simulink model "DemonstratorSimscape"  (R2020b)
settings: Solver=ode113  StartTime=0.0  StopTime=t_stop*0+20  FixedStep=1e-4
values from neighbouring files (symbols this model uses):
  brkD = 0    [main.m]
  brkI = 1e4    (= 10000)    [main.m]
  brkP = 1e5    (= 100000)    [main.m]
  d_drm = 0.5*d_drum    [main.m]
  d_shm = 0.4*d_sheave    [main.m]
  DeltaCable0 = 0    [main.m]
  Droop_scaling = 0    [main.m]
  eta_sh = 0.015    [main.m]
  filt_NUM = ones(1,200)*0.005    [main.m]
  g = 9.80665    [main.m]
  Iw = 0.5*(W.i + M.in*GB.r^2)    [main.m]
  Kp_mul = 0.3    [main.m]
  Lc0 = abs((T.ph-L.height-P.d-L.z0)*0.001)    [main.m]
  Ls1 = ((T.ph-0.5*W.pd)/1000)    [main.m]
  Ls2 = ((0.5*(T.s2+P.d)-2*P.d)/1000)    [main.m]
  M = 50e3    (= 50000)    [calcGrav.m]
  phi0_drm = -90    [main.m]
  phi0_shm = -90    [main.m]
  r_sheave = P.d*0.5    [main.m]
  s = tf('s')    [calcGrav.m]
  tau_brk = 0.001    [main.m]
  tau_em = 60e-3    (= 0.06)    [calcGrav.m]    (also in main.m)
  tau_m = tau_w/GB.r    [main.m]
  Tmax = 400e3    (= 400000)    [main.m]
  Tn_mul = 10    [main.m]
  x_drm = 0.7*r_drum    [main.m]
  x_shm = 0.7*r_sheave    [main.m]
  z0 = 0    [calcGrav.m]    (also in main.m = L.z0-P.d*0.5-P.d-P.d-L.height-T.h1-T.h2-32)
undefined symbols (not defined in the file or in its folder): C, CA, Controller_sampleTime, DiscIntNeverNeededParam, GB, L, P, Part, T, VFD_acceleration_model_factor, VFD_Adapt_factor_lower_p1458, VFD_Adapt_factor_upper_p1459, VFD_Curr_limit_var_p0641, VFD_Current_limit_p0640, VFD_Id_setp_total_r1624, VFD_Iq, VFD_Kp_n_basic_p1460, VFD_M, VFD_M_accel_T_smooth_p1517, VFD_M_lim_var_fixS_src_p1551, VFD_M_max_lower_p1521, VFD_M_max_lower_scal_p1525, VFD_M_max_up_mot_scal_p1524, VFD_M_max_upper_p1520, VFD_n_act_T_smooth_p1442, VFD_n_ctr_Kp_n_up_scal_p1461, VFD_n_ctr_Tn_n_up_sca_p1463, VFD_n_ctrl_adapt_Kp_lower_p1456, VFD_n_ctrl_adapt_Kp_upper_p1457, VFD_n_ctrl_Adpt_sig_Kp_p1455, VFD_n_ctrl_Kp_scal_p1466, VFD_n_ctrl_n_lower_p1464, VFD_n_ctrl_n_upper_p1465, VFD_n_ctrl_Tn_n_lower_p1462, VFD_n_limit_neg_p1086, VFD_n_limit_pos_p1083, VFD_n_limit_setp_p1063, VFD_n_max_p1082, VFD_n_set_filt_1_T_p1416, VFD_P_max_gen_p1531, VFD_P_max_mot_p1530, VFD_PU_I_outp_max_r0289, VFD_RFG_ramp_down_time_p1121, VFD_RFG_ramp_up_time_p1120, VFD_RFG_t_RD_scal_p1139, VFD_RFG_t_RU_scal_p1138, VSD, W, X, Y, Z
libraries: sm_lib x248, nesl_utility x128, simulink x49, pid_lib x4, cstblocks x2, simulink_extras x2
(part 7 of 10)

== system DemonstratorSimscape/Transmission System/Anchor and Load/Sheave_03/Sheave3 ==
  Rigid Transform : sm_lib/Frames and Transforms/Rigid Transform  TranslationMethod=None  TranslationStandardOffset=0  TranslationLengthUnit=m  TranslationStandardAxis=+Z  TranslationCartesianOffset=[0 0 0]  TranslationROffset=0  TranslationROffsetUnits=m  TranslationZOffset=0  TranslationZOffsetUnits=m  TranslationThetaOffset=0  TranslationThetaOffsetUnits=deg  RotationMethod=StandardAxis  RotationAngleUnits=deg  RotationStandardAxis=+X  RotationAngle=90  RotationArbitraryAxis=[0 0 1]  FollAlignAxisA=+X  BaseAlignAxisA=+Y  FollAlignAxisB=+Y  BaseAlignAxisB=+Z  RotationSequenceAxes=FollowerAxes  RotationSequence=XYX  RotationSequenceAngles=[0 0 0]  RotationSequenceAnglesUnits=deg  RotationMatrix=[1 0 0; 0 1 0; 0 0 1]
  pulley1 : sm_lib/Body Elements/Cylindrical Solid  GraphicAmbientColor=[0.15 0.15 0.15 1.0]  BasedOnType=Mass  CenterOfMass=[0 0 0]  CenterOfMassUnits=m  GraphicDiffuseColor=c.sheave  CylinderLength=P.h  CylinderLengthUnits=mm  CylinderRadius=P.d*0.5  CylinderRadiusUnits=mm  Density=0  DensityUnits=kg/m^3  DoExposeReferenceFrame=off  GraphicEmissiveColor=[0.0 0.0 0.0 1.0]  ExportEntireGeometry=off  SerializedFrames=<Frames><Frame><Id>Frame1</Id><Value><Name>F1</Name><Origin><Source>ReferenceFrame</Source><FeatureName></FeatureName></Origin><PrimaryAxis><DefinedDirection>+Z</DefinedDirection><Source>ReferenceFrame</Source><SourceDirection>-Y</SourceDirection><FeatureName></FeatureName></PrimaryAxis><SecondaryAxis><DefinedDirection>+X</DefinedDirection><Source>ReferenceFrame</Source><SourceDirection>+X</SourceDirection><FeatureName></FeatureName></SecondaryAxis></Value></Frame></Frames>  MarkerShape=Frame  MarkerSize=10  GraphicType=FromGeometry  InertiaType=CalculateFromGeometry  Mass=P.m  MassUnits=kg  MomentsOfInertia=[1 1 1]  MomentsOfInertiaUnits=kg*m^2  GraphicOpacity=1.0  ProductsOfInertia=[0 0 0]  ProductsOfInertiaUnits=kg*m^2  GraphicShininess=10  GraphicSpecularColor=[0.8 0.8 0.8]  GraphicVisPropType=SimpleVisualProperties
  tags : Subsystem  mask{phi0=phi0_shm, s=-1}
      mask prompts: phi0 "angle (deg)"; s "direction (1 | -1)"
  F : PMIOPort  Side=Left
  R : PMIOPort  Port=2  Side=Right
  connections:
  R/RConn1 -- tags/LConn1 -- Rigid Transform/RConn1 -- F/RConn1
  pulley1/LConn1 -- Rigid Transform/LConn1

== system DemonstratorSimscape/Transmission System/Anchor and Load/Sheave_05/Bending loss ==
  Sin (kN) : Inport
  w (deg/s) : Inport  Port=2
  Add : Sum
  Add1 : Sum  Inputs=+-
  Constant : Constant
  Constant2 : Constant
  Math Function : Math  Operator=pow  SignedPower=on  SaturateOnIntegerOverflow=on
  Product : Product
  Product1 : Product
  Scope : Scope
  dT_Gain : Gain  Gain=0
  dr for positive omega : Constant  Value=-1
  dr switch : MATLAB Function  TreatAsAtomicUnit=on
  eta_sh : Constant  Value=eta_sh
  torque (Nm) : Gain  Gain=r_sheave
  dT (Nm) : Outport  VectorParamsAs1DForOutWhenUnconnected=off
  Sout (kN) : Outport  Port=2  VectorParamsAs1DForOutWhenUnconnected=off
  wires:
  Add/1 -> Math Function/1
  Sin (kN)/1 -> Product1/2, Product/2
  torque (Nm)/1 -> Scope/1, dT_Gain/1
  Math Function/1 -> Add1/1, Product1/1
  Add1/1 -> Product/1
  Product/1 -> torque (Nm)/1
  eta_sh/1 -> Add/2
  Constant/1 -> Add/1
  Constant2/1 -> Add1/2
  Product1/1 -> Sout (kN)/1
  dT_Gain/1 -> dT (Nm)/1
  dr for positive omega/1 -> dr switch/2(dr_wpos)
  dr switch/1(dr) -> Math Function/2
  w (deg/s)/1 -> dr switch/1(w)

== system DemonstratorSimscape/Transmission System/Anchor and Load/Sheave_05/PS>Sim2 ==
  b (deg/s^2) : nesl_utility/PS-Simulink Converter  PhysicalDomain=network_engine_domain  SubClassName=ps_output  LeftPortType=input  RightPortType=output  PseudoPeriodic=off  Frequencies=[]  Unit=deg/s^2  AffineConversion=off
  fc (N) : nesl_utility/PS-Simulink Converter  PhysicalDomain=network_engine_domain  SubClassName=ps_output  LeftPortType=input  RightPortType=output  PseudoPeriodic=off  Frequencies=[]  Unit=N  AffineConversion=off
  ft (N) : nesl_utility/PS-Simulink Converter  PhysicalDomain=network_engine_domain  SubClassName=ps_output  LeftPortType=input  RightPortType=output  PseudoPeriodic=off  Frequencies=[]  Unit=N  AffineConversion=off
  q (deg) : nesl_utility/PS-Simulink Converter  PhysicalDomain=network_engine_domain  SubClassName=ps_output  LeftPortType=input  RightPortType=output  PseudoPeriodic=off  Frequencies=[]  Unit=deg  AffineConversion=off
  t (Nm) : nesl_utility/PS-Simulink Converter  PhysicalDomain=network_engine_domain  SubClassName=ps_output  LeftPortType=input  RightPortType=output  PseudoPeriodic=off  Frequencies=[]  Unit=N*m  AffineConversion=off
  tc (Nm) : nesl_utility/PS-Simulink Converter  PhysicalDomain=network_engine_domain  SubClassName=ps_output  LeftPortType=input  RightPortType=output  PseudoPeriodic=off  Frequencies=[]  Unit=N*m  AffineConversion=off
  tt (Nm) : nesl_utility/PS-Simulink Converter  PhysicalDomain=network_engine_domain  SubClassName=ps_output  LeftPortType=input  RightPortType=output  PseudoPeriodic=off  Frequencies=[]  Unit=N*m  AffineConversion=off
  w (deg/s) : nesl_utility/PS-Simulink Converter  PhysicalDomain=network_engine_domain  SubClassName=ps_output  LeftPortType=input  RightPortType=output  PseudoPeriodic=off  Frequencies=[]  Unit=deg/s  AffineConversion=off
  q : PMIOPort  Side=Left
  Conn2 : PMIOPort  Port=2  Side=Left
  Conn3 : PMIOPort  Port=3  Side=Left
  Conn4 : PMIOPort  Port=4  Side=Left
  Conn5 : PMIOPort  Port=5  Side=Left
  Conn6 : PMIOPort  Port=6  Side=Left
  Conn7 : PMIOPort  Port=7  Side=Left
  Conn8 : PMIOPort  Port=8  Side=Left
  Out1 : Outport  VectorParamsAs1DForOutWhenUnconnected=off
  Out2 : Outport  Port=2  VectorParamsAs1DForOutWhenUnconnected=off
  Out3 : Outport  Port=3  VectorParamsAs1DForOutWhenUnconnected=off
  Out4 : Outport  Port=4  VectorParamsAs1DForOutWhenUnconnected=off
  Out5 : Outport  Port=5  VectorParamsAs1DForOutWhenUnconnected=off
  Out6 : Outport  Port=6  VectorParamsAs1DForOutWhenUnconnected=off
  Out7 : Outport  Port=7  VectorParamsAs1DForOutWhenUnconnected=off
  Out8 : Outport  Port=8  VectorParamsAs1DForOutWhenUnconnected=off
  wires:
  tt (Nm)/1 -> Out8/1
  ft (N)/1 -> Out7/1
  tc (Nm)/1 -> Out6/1
  fc (N)/1 -> Out5/1
  t (Nm)/1 -> Out4/1
  b (deg/s^2)/1 -> Out3/1
  w (deg/s)/1 -> Out2/1
  q (deg)/1 -> Out1/1
  connections:
  Conn8/RConn1 -- tt (Nm)/LConn1
  ft (N)/LConn1 -- Conn7/RConn1
  Conn6/RConn1 -- tc (Nm)/LConn1
  fc (N)/LConn1 -- Conn5/RConn1
  Conn4/RConn1 -- t (Nm)/LConn1
  Conn3/RConn1 -- b (deg/s^2)/LConn1
  Conn2/RConn1 -- w (deg/s)/LConn1
  q/RConn1 -- q (deg)/LConn1

== system DemonstratorSimscape/Transmission System/Anchor and Load/Sheave_05/Sheave5 ==
  Rigid Transform : sm_lib/Frames and Transforms/Rigid Transform  TranslationMethod=None  TranslationStandardOffset=0  TranslationLengthUnit=m  TranslationStandardAxis=+Z  TranslationCartesianOffset=[0 0 0]  TranslationROffset=0  TranslationROffsetUnits=m  TranslationZOffset=0  TranslationZOffsetUnits=m  TranslationThetaOffset=0  TranslationThetaOffsetUnits=deg  RotationMethod=StandardAxis  RotationAngleUnits=deg  RotationStandardAxis=+X  RotationAngle=90  RotationArbitraryAxis=[0 0 1]  FollAlignAxisA=+X  BaseAlignAxisA=+Y  FollAlignAxisB=+Y  BaseAlignAxisB=+Z  RotationSequenceAxes=FollowerAxes  RotationSequence=XYX  RotationSequenceAngles=[0 0 0]  RotationSequenceAnglesUnits=deg  RotationMatrix=[1 0 0; 0 1 0; 0 0 1]
  pulley2 : sm_lib/Body Elements/Cylindrical Solid  GraphicAmbientColor=[0.15 0.15 0.15 1.0]  BasedOnType=Mass  CenterOfMass=[0 0 0]  CenterOfMassUnits=m  GraphicDiffuseColor=c.sheave  CylinderLength=P.h  CylinderLengthUnits=mm  CylinderRadius=P.d*0.5  CylinderRadiusUnits=mm  Density=0  DensityUnits=kg/m^3  DoExposeReferenceFrame=off  GraphicEmissiveColor=[0.0 0.0 0.0 1.0]  ExportEntireGeometry=off  SerializedFrames=<Frames><Frame><Id>Frame1</Id><Value><Name>F1</Name><Origin><Source>ReferenceFrame</Source><FeatureName></FeatureName></Origin><PrimaryAxis><DefinedDirection>+Z</DefinedDirection><Source>ReferenceFrame</Source><SourceDirection>-Y</SourceDirection><FeatureName></FeatureName></PrimaryAxis><SecondaryAxis><DefinedDirection>+X</DefinedDirection><Source>ReferenceFrame</Source><SourceDirection>+X</SourceDirection><FeatureName></FeatureName></SecondaryAxis></Value></Frame></Frames>  MarkerShape=Frame  MarkerSize=10  GraphicType=FromGeometry  InertiaType=CalculateFromGeometry  Mass=P.m  MassUnits=kg  MomentsOfInertia=[1 1 1]  MomentsOfInertiaUnits=kg*m^2  GraphicOpacity=1.0  ProductsOfInertia=[0 0 0]  ProductsOfInertiaUnits=kg*m^2  GraphicShininess=10  GraphicSpecularColor=[0.8 0.8 0.8]  GraphicVisPropType=SimpleVisualProperties
  tags : Subsystem  mask{phi0=phi0_shm, s=-1}
      mask prompts: phi0 "angle (deg)"; s "direction (1 | -1)"
  F : PMIOPort  Side=Left
  R : PMIOPort  Port=2  Side=Right
  connections:
  R/RConn1 -- tags/LConn1 -- Rigid Transform/RConn1 -- F/RConn1
  pulley2/LConn1 -- Rigid Transform/LConn1

== system DemonstratorSimscape/Transmission System/Roof Pulley Set/Sheave_01/Bending loss ==
  Sin (kN) : Inport
  w (deg/s) : Inport  Port=2
  Add : Sum
  Add1 : Sum  Inputs=+-
  Constant : Constant
  Constant2 : Constant
  Math Function : Math  Operator=pow  SignedPower=on  SaturateOnIntegerOverflow=on
  Product : Product
  Product1 : Product
  Scope : Scope
  dT_Gain : Gain
  dr for positive omega : Constant  Value=-1
  dr switch : MATLAB Function  TreatAsAtomicUnit=on
  eta_sh : Constant  Value=eta_sh/2
  torque (Nm) : Gain  Gain=r_sheave
  dT (Nm) : Outport  VectorParamsAs1DForOutWhenUnconnected=off
  Sout (kN) : Outport  Port=2  VectorParamsAs1DForOutWhenUnconnected=off
  wires:
  Add/1 -> Math Function/1
  Sin (kN)/1 -> Product1/2, Product/2
  torque (Nm)/1 -> Scope/1, dT_Gain/1
  Math Function/1 -> Add1/1, Product1/1
  Add1/1 -> Product/1
  Product/1 -> torque (Nm)/1
  eta_sh/1 -> Add/2
  Constant/1 -> Add/1
  Constant2/1 -> Add1/2
  Product1/1 -> Sout (kN)/1
  dT_Gain/1 -> dT (Nm)/1
  dr for positive omega/1 -> dr switch/2(dr_wpos)
  dr switch/1(dr) -> Math Function/2
  w (deg/s)/1 -> dr switch/1(w)

== system DemonstratorSimscape/Transmission System/Roof Pulley Set/Sheave_01/PS>Sim1 ==
  b (deg/s^2) : nesl_utility/PS-Simulink Converter  PhysicalDomain=network_engine_domain  SubClassName=ps_output  LeftPortType=input  RightPortType=output  PseudoPeriodic=off  Frequencies=[]  Unit=deg/s^2  AffineConversion=off
  fc (N) : nesl_utility/PS-Simulink Converter  PhysicalDomain=network_engine_domain  SubClassName=ps_output  LeftPortType=input  RightPortType=output  PseudoPeriodic=off  Frequencies=[]  Unit=N  AffineConversion=off
  ft (N) : nesl_utility/PS-Simulink Converter  PhysicalDomain=network_engine_domain  SubClassName=ps_output  LeftPortType=input  RightPortType=output  PseudoPeriodic=off  Frequencies=[]  Unit=N  AffineConversion=off
  q (deg) : nesl_utility/PS-Simulink Converter  PhysicalDomain=network_engine_domain  SubClassName=ps_output  LeftPortType=input  RightPortType=output  PseudoPeriodic=off  Frequencies=[]  Unit=deg  AffineConversion=off
  t (Nm) : nesl_utility/PS-Simulink Converter  PhysicalDomain=network_engine_domain  SubClassName=ps_output  LeftPortType=input  RightPortType=output  PseudoPeriodic=off  Frequencies=[]  Unit=N*m  AffineConversion=off
  tc (Nm) : nesl_utility/PS-Simulink Converter  PhysicalDomain=network_engine_domain  SubClassName=ps_output  LeftPortType=input  RightPortType=output  PseudoPeriodic=off  Frequencies=[]  Unit=N*m  AffineConversion=off
  tt (Nm) : nesl_utility/PS-Simulink Converter  PhysicalDomain=network_engine_domain  SubClassName=ps_output  LeftPortType=input  RightPortType=output  PseudoPeriodic=off  Frequencies=[]  Unit=N*m  AffineConversion=off
  w (deg/s) : nesl_utility/PS-Simulink Converter  PhysicalDomain=network_engine_domain  SubClassName=ps_output  LeftPortType=input  RightPortType=output  PseudoPeriodic=off  Frequencies=[]  Unit=deg/s  AffineConversion=off
  q : PMIOPort  Side=Left
  Conn2 : PMIOPort  Port=2  Side=Left
  Conn3 : PMIOPort  Port=3  Side=Left
  Conn4 : PMIOPort  Port=4  Side=Left
  Conn5 : PMIOPort  Port=5  Side=Left
  Conn6 : PMIOPort  Port=6  Side=Left
  Conn7 : PMIOPort  Port=7  Side=Left
  Conn8 : PMIOPort  Port=8  Side=Left
  Out1 : Outport  VectorParamsAs1DForOutWhenUnconnected=off
  Out2 : Outport  Port=2  VectorParamsAs1DForOutWhenUnconnected=off
  Out3 : Outport  Port=3  VectorParamsAs1DForOutWhenUnconnected=off
  Out4 : Outport  Port=4  VectorParamsAs1DForOutWhenUnconnected=off
  Out5 : Outport  Port=5  VectorParamsAs1DForOutWhenUnconnected=off
  Out6 : Outport  Port=6  VectorParamsAs1DForOutWhenUnconnected=off
  Out7 : Outport  Port=7  VectorParamsAs1DForOutWhenUnconnected=off
  Out8 : Outport  Port=8  VectorParamsAs1DForOutWhenUnconnected=off
  wires:
  q (deg)/1 -> Out1/1
  w (deg/s)/1 -> Out2/1
  b (deg/s^2)/1 -> Out3/1
  t (Nm)/1 -> Out4/1
  fc (N)/1 -> Out5/1
  tc (Nm)/1 -> Out6/1
  ft (N)/1 -> Out7/1
  tt (Nm)/1 -> Out8/1
  connections:
  q/RConn1 -- q (deg)/LConn1
  Conn2/RConn1 -- w (deg/s)/LConn1
  Conn3/RConn1 -- b (deg/s^2)/LConn1
  Conn4/RConn1 -- t (Nm)/LConn1
  fc (N)/LConn1 -- Conn5/RConn1
  Conn6/RConn1 -- tc (Nm)/LConn1
  ft (N)/LConn1 -- Conn7/RConn1
  Conn8/RConn1 -- tt (Nm)/LConn1

== system DemonstratorSimscape/Transmission System/Roof Pulley Set/Sheave_01/Sheave1 ==
  Rigid Transform : sm_lib/Frames and Transforms/Rigid Transform  TranslationMethod=None  TranslationStandardOffset=0  TranslationLengthUnit=m  TranslationStandardAxis=+Z  TranslationCartesianOffset=[0 0 0]  TranslationROffset=0  TranslationROffsetUnits=m  TranslationZOffset=0  TranslationZOffsetUnits=m  TranslationThetaOffset=0  TranslationThetaOffsetUnits=deg  RotationMethod=StandardAxis  RotationAngleUnits=deg  RotationStandardAxis=+X  RotationAngle=90  RotationArbitraryAxis=[0 0 1]  FollAlignAxisA=+X  BaseAlignAxisA=+Y  FollAlignAxisB=+Y  BaseAlignAxisB=+Z  RotationSequenceAxes=FollowerAxes  RotationSequence=XYX  RotationSequenceAngles=[0 0 0]  RotationSequenceAnglesUnits=deg  RotationMatrix=[1 0 0; 0 1 0; 0 0 1]
  pulley2 : sm_lib/Body Elements/Cylindrical Solid  GraphicAmbientColor=[0.15 0.15 0.15 1.0]  BasedOnType=Mass  CenterOfMass=[0 0 0]  CenterOfMassUnits=m  GraphicDiffuseColor=c.sheave  CylinderLength=P.h  CylinderLengthUnits=mm  CylinderRadius=P.d*0.5  CylinderRadiusUnits=mm  Density=L.den  DensityUnits=g/cm^3  DoExposeReferenceFrame=off  GraphicEmissiveColor=[0.0 0.0 0.0 1.0]  ExportEntireGeometry=off  SerializedFrames=<Frames><Frame><Id>Frame1</Id><Value><Name>F1</Name><Origin><Source>ReferenceFrame</Source><FeatureName></FeatureName></Origin><PrimaryAxis><DefinedDirection>+Z</DefinedDirection><Source>ReferenceFrame</Source><SourceDirection>-Y</SourceDirection><FeatureName></FeatureName></PrimaryAxis><SecondaryAxis><DefinedDirection>+X</DefinedDirection><Source>ReferenceFrame</Source><SourceDirection>+X</SourceDirection><FeatureName></FeatureName></SecondaryAxis></Value></Frame></Frames>  MarkerShape=Frame  MarkerSize=10  GraphicType=FromGeometry  InertiaType=CalculateFromGeometry  Mass=P.m  MassUnits=kg  MomentsOfInertia=[1 1 1]  MomentsOfInertiaUnits=kg*m^2  GraphicOpacity=1.0  ProductsOfInertia=[0 0 0]  ProductsOfInertiaUnits=kg*m^2  GraphicShininess=10  GraphicSpecularColor=[0.8 0.8 0.8]  GraphicVisPropType=SimpleVisualProperties
  tags : Subsystem  mask{phi0=phi0_shm, s=1}
      mask prompts: phi0 "angle (deg)"; s "direction (1 | -1)"
  F : PMIOPort  Side=Left
  R : PMIOPort  Port=2  Side=Right
  connections:
  R/RConn1 -- tags/LConn1 -- Rigid Transform/RConn1 -- F/RConn1
  pulley2/LConn1 -- Rigid Transform/LConn1

== system DemonstratorSimscape/Transmission System/Roof Pulley Set/Sheave_02/Bending loss ==
  Sin (kN) : Inport
  w (deg/s) : Inport  Port=2
  Add : Sum
  Add1 : Sum  Inputs=+-
  Constant : Constant
  Constant2 : Constant
  Math Function : Math  Operator=pow  SignedPower=on  SaturateOnIntegerOverflow=on
  Product : Product
  Product1 : Product
  Scope : Scope
  dT_Gain : Gain
  dr for positive omega : Constant  Value=-1
  dr switch : MATLAB Function  TreatAsAtomicUnit=on
  eta_sh : Constant  Value=eta_sh/2
  torque (Nm) : Gain  Gain=r_sheave
  dT (Nm) : Outport  VectorParamsAs1DForOutWhenUnconnected=off
  Sout (kN) : Outport  Port=2  VectorParamsAs1DForOutWhenUnconnected=off
  wires:
  Add/1 -> Math Function/1
  Sin (kN)/1 -> Product1/2, Product/2
  torque (Nm)/1 -> Scope/1, dT_Gain/1
  Math Function/1 -> Add1/1, Product1/1
  Add1/1 -> Product/1
  Product/1 -> torque (Nm)/1
  eta_sh/1 -> Add/2
  Constant/1 -> Add/1
  Constant2/1 -> Add1/2
  Product1/1 -> Sout (kN)/1
  dT_Gain/1 -> dT (Nm)/1
  dr for positive omega/1 -> dr switch/2(dr_wpos)
  dr switch/1(dr) -> Math Function/2
  w (deg/s)/1 -> dr switch/1(w)

== system DemonstratorSimscape/Transmission System/Roof Pulley Set/Sheave_02/PS>Sim1 ==
  b (deg/s^2) : nesl_utility/PS-Simulink Converter  PhysicalDomain=network_engine_domain  SubClassName=ps_output  LeftPortType=input  RightPortType=output  PseudoPeriodic=off  Frequencies=[]  Unit=deg/s^2  AffineConversion=off
  fc (N) : nesl_utility/PS-Simulink Converter  PhysicalDomain=network_engine_domain  SubClassName=ps_output  LeftPortType=input  RightPortType=output  PseudoPeriodic=off  Frequencies=[]  Unit=N  AffineConversion=off
  ft (N) : nesl_utility/PS-Simulink Converter  PhysicalDomain=network_engine_domain  SubClassName=ps_output  LeftPortType=input  RightPortType=output  PseudoPeriodic=off  Frequencies=[]  Unit=N  AffineConversion=off
  q (deg) : nesl_utility/PS-Simulink Converter  PhysicalDomain=network_engine_domain  SubClassName=ps_output  LeftPortType=input  RightPortType=output  PseudoPeriodic=off  Frequencies=[]  Unit=deg  AffineConversion=off
  t (Nm) : nesl_utility/PS-Simulink Converter  PhysicalDomain=network_engine_domain  SubClassName=ps_output  LeftPortType=input  RightPortType=output  PseudoPeriodic=off  Frequencies=[]  Unit=N*m  AffineConversion=off
  tc (Nm) : nesl_utility/PS-Simulink Converter  PhysicalDomain=network_engine_domain  SubClassName=ps_output  LeftPortType=input  RightPortType=output  PseudoPeriodic=off  Frequencies=[]  Unit=N*m  AffineConversion=off
  tt (Nm) : nesl_utility/PS-Simulink Converter  PhysicalDomain=network_engine_domain  SubClassName=ps_output  LeftPortType=input  RightPortType=output  PseudoPeriodic=off  Frequencies=[]  Unit=N*m  AffineConversion=off
  w (deg/s) : nesl_utility/PS-Simulink Converter  PhysicalDomain=network_engine_domain  SubClassName=ps_output  LeftPortType=input  RightPortType=output  PseudoPeriodic=off  Frequencies=[]  Unit=deg/s  AffineConversion=off
  q : PMIOPort  Side=Left
  Conn2 : PMIOPort  Port=2  Side=Left
  Conn3 : PMIOPort  Port=3  Side=Left
  Conn4 : PMIOPort  Port=4  Side=Left
  Conn5 : PMIOPort  Port=5  Side=Left
  Conn6 : PMIOPort  Port=6  Side=Left
  Conn7 : PMIOPort  Port=7  Side=Left
  Conn8 : PMIOPort  Port=8  Side=Left
  Out1 : Outport  VectorParamsAs1DForOutWhenUnconnected=off
  Out2 : Outport  Port=2  VectorParamsAs1DForOutWhenUnconnected=off
  Out3 : Outport  Port=3  VectorParamsAs1DForOutWhenUnconnected=off
  Out4 : Outport  Port=4  VectorParamsAs1DForOutWhenUnconnected=off
  Out5 : Outport  Port=5  VectorParamsAs1DForOutWhenUnconnected=off
  Out6 : Outport  Port=6  VectorParamsAs1DForOutWhenUnconnected=off
  Out7 : Outport  Port=7  VectorParamsAs1DForOutWhenUnconnected=off
  Out8 : Outport  Port=8  VectorParamsAs1DForOutWhenUnconnected=off
  wires:
  tt (Nm)/1 -> Out8/1
  ft (N)/1 -> Out7/1
  tc (Nm)/1 -> Out6/1
  fc (N)/1 -> Out5/1
  t (Nm)/1 -> Out4/1
  b (deg/s^2)/1 -> Out3/1
  w (deg/s)/1 -> Out2/1
  q (deg)/1 -> Out1/1
  connections:
  Conn8/RConn1 -- tt (Nm)/LConn1
  ft (N)/LConn1 -- Conn7/RConn1
  Conn6/RConn1 -- tc (Nm)/LConn1
  fc (N)/LConn1 -- Conn5/RConn1
  Conn4/RConn1 -- t (Nm)/LConn1
  Conn3/RConn1 -- b (deg/s^2)/LConn1
  Conn2/RConn1 -- w (deg/s)/LConn1
  q/RConn1 -- q (deg)/LConn1

== system DemonstratorSimscape/Transmission System/Roof Pulley Set/Sheave_02/Sheave2 ==
  Rigid Transform : sm_lib/Frames and Transforms/Rigid Transform  TranslationMethod=None  TranslationStandardOffset=0  TranslationLengthUnit=m  TranslationStandardAxis=+Z  TranslationCartesianOffset=[0 0 0]  TranslationROffset=0  TranslationROffsetUnits=m  TranslationZOffset=0  TranslationZOffsetUnits=m  TranslationThetaOffset=0  TranslationThetaOffsetUnits=deg  RotationMethod=StandardAxis  RotationAngleUnits=deg  RotationStandardAxis=+X  RotationAngle=90  RotationArbitraryAxis=[0 0 1]  FollAlignAxisA=+X  BaseAlignAxisA=+Y  FollAlignAxisB=+Y  BaseAlignAxisB=+Z  RotationSequenceAxes=FollowerAxes  RotationSequence=XYX  RotationSequenceAngles=[0 0 0]  RotationSequenceAnglesUnits=deg  RotationMatrix=[1 0 0; 0 1 0; 0 0 1]
  pulley2 : sm_lib/Body Elements/Cylindrical Solid  GraphicAmbientColor=[0.15 0.15 0.15 1.0]  BasedOnType=Mass  CenterOfMass=[0 0 0]  CenterOfMassUnits=m  GraphicDiffuseColor=c.sheave  CylinderLength=P.h  CylinderLengthUnits=mm  CylinderRadius=P.d*0.5  CylinderRadiusUnits=mm  Density=0  DensityUnits=kg/m^3  DoExposeReferenceFrame=off  GraphicEmissiveColor=[0.0 0.0 0.0 1.0]  ExportEntireGeometry=off  SerializedFrames=<Frames><Frame><Id>Frame1</Id><Value><Name>F1</Name><Origin><Source>ReferenceFrame</Source><FeatureName></FeatureName></Origin><PrimaryAxis><DefinedDirection>+Z</DefinedDirection><Source>ReferenceFrame</Source><SourceDirection>-Y</SourceDirection><FeatureName></FeatureName></PrimaryAxis><SecondaryAxis><DefinedDirection>+X</DefinedDirection><Source>ReferenceFrame</Source><SourceDirection>+X</SourceDirection><FeatureName></FeatureName></SecondaryAxis></Value></Frame></Frames>  MarkerShape=Frame  MarkerSize=10  GraphicType=FromGeometry  InertiaType=CalculateFromGeometry  Mass=P.m  MassUnits=kg  MomentsOfInertia=[1 1 1]  MomentsOfInertiaUnits=kg*m^2  GraphicOpacity=1.0  ProductsOfInertia=[0 0 0]  ProductsOfInertiaUnits=kg*m^2  GraphicShininess=10  GraphicSpecularColor=[0.8 0.8 0.8]  GraphicVisPropType=SimpleVisualProperties
  tags : Subsystem  mask{phi0=phi0_shm, s=1}
      mask prompts: phi0 "angle (deg)"; s "direction (1 | -1)"
  F : PMIOPort  Side=Left
  R : PMIOPort  Port=2  Side=Right
  connections:
  R/RConn1 -- Rigid Transform/RConn1 -- tags/LConn1 -- F/RConn1
  pulley2/LConn1 -- Rigid Transform/LConn1

== system DemonstratorSimscape/Transmission System/Roof Pulley Set/Sheave_04/PS>Sim1 ==
  b (deg/s^2) : nesl_utility/PS-Simulink Converter  PhysicalDomain=network_engine_domain  SubClassName=ps_output  LeftPortType=input  RightPortType=output  PseudoPeriodic=off  Frequencies=[]  Unit=deg/s^2  AffineConversion=off
  fc (N) : nesl_utility/PS-Simulink Converter  PhysicalDomain=network_engine_domain  SubClassName=ps_output  LeftPortType=input  RightPortType=output  PseudoPeriodic=off  Frequencies=[]  Unit=N  AffineConversion=off
  ft (N) : nesl_utility/PS-Simulink Converter  PhysicalDomain=network_engine_domain  SubClassName=ps_output  LeftPortType=input  RightPortType=output  PseudoPeriodic=off  Frequencies=[]  Unit=N  AffineConversion=off
  q (deg) : nesl_utility/PS-Simulink Converter  PhysicalDomain=network_engine_domain  SubClassName=ps_output  LeftPortType=input  RightPortType=output  PseudoPeriodic=off  Frequencies=[]  Unit=deg  AffineConversion=off
  t (Nm) : nesl_utility/PS-Simulink Converter  PhysicalDomain=network_engine_domain  SubClassName=ps_output  LeftPortType=input  RightPortType=output  PseudoPeriodic=off  Frequencies=[]  Unit=N*m  AffineConversion=off
  tc (Nm) : nesl_utility/PS-Simulink Converter  PhysicalDomain=network_engine_domain  SubClassName=ps_output  LeftPortType=input  RightPortType=output  PseudoPeriodic=off  Frequencies=[]  Unit=N*m  AffineConversion=off
  tt (Nm) : nesl_utility/PS-Simulink Converter  PhysicalDomain=network_engine_domain  SubClassName=ps_output  LeftPortType=input  RightPortType=output  PseudoPeriodic=off  Frequencies=[]  Unit=N*m  AffineConversion=off
  w (deg/s) : nesl_utility/PS-Simulink Converter  PhysicalDomain=network_engine_domain  SubClassName=ps_output  LeftPortType=input  RightPortType=output  PseudoPeriodic=off  Frequencies=[]  Unit=deg/s  AffineConversion=off
  q : PMIOPort  Side=Left
  Conn2 : PMIOPort  Port=2  Side=Left
  Conn3 : PMIOPort  Port=3  Side=Left
  Conn4 : PMIOPort  Port=4  Side=Left
  Conn5 : PMIOPort  Port=5  Side=Left
  Conn6 : PMIOPort  Port=6  Side=Left
  Conn7 : PMIOPort  Port=7  Side=Left
  Conn8 : PMIOPort  Port=8  Side=Left
  Out1 : Outport  VectorParamsAs1DForOutWhenUnconnected=off
  Out2 : Outport  Port=2  VectorParamsAs1DForOutWhenUnconnected=off
  Out3 : Outport  Port=3  VectorParamsAs1DForOutWhenUnconnected=off
  Out4 : Outport  Port=4  VectorParamsAs1DForOutWhenUnconnected=off
  Out5 : Outport  Port=5  VectorParamsAs1DForOutWhenUnconnected=off
  Out6 : Outport  Port=6  VectorParamsAs1DForOutWhenUnconnected=off
  Out7 : Outport  Port=7  VectorParamsAs1DForOutWhenUnconnected=off
  Out8 : Outport  Port=8  VectorParamsAs1DForOutWhenUnconnected=off
  wires:
  q (deg)/1 -> Out1/1
  w (deg/s)/1 -> Out2/1
  b (deg/s^2)/1 -> Out3/1
  t (Nm)/1 -> Out4/1
  fc (N)/1 -> Out5/1
  tc (Nm)/1 -> Out6/1
  ft (N)/1 -> Out7/1
  tt (Nm)/1 -> Out8/1
  connections:
  q/RConn1 -- q (deg)/LConn1
  Conn2/RConn1 -- w (deg/s)/LConn1
  Conn3/RConn1 -- b (deg/s^2)/LConn1
  Conn4/RConn1 -- t (Nm)/LConn1
  fc (N)/LConn1 -- Conn5/RConn1
  Conn6/RConn1 -- tc (Nm)/LConn1
  ft (N)/LConn1 -- Conn7/RConn1
  Conn8/RConn1 -- tt (Nm)/LConn1

== system DemonstratorSimscape/Transmission System/Roof Pulley Set/Sheave_04/Pulley rught red2 ==
  Rigid Transform : sm_lib/Frames and Transforms/Rigid Transform  TranslationMethod=None  TranslationStandardOffset=0  TranslationLengthUnit=m  TranslationStandardAxis=+Z  TranslationCartesianOffset=[0 0 0]  TranslationROffset=0  TranslationROffsetUnits=m  TranslationZOffset=0  TranslationZOffsetUnits=m  TranslationThetaOffset=0  TranslationThetaOffsetUnits=deg  RotationMethod=StandardAxis  RotationAngleUnits=deg  RotationStandardAxis=+X  RotationAngle=90  RotationArbitraryAxis=[0 0 1]  FollAlignAxisA=+X  BaseAlignAxisA=+Y  FollAlignAxisB=+Y  BaseAlignAxisB=+Z  RotationSequenceAxes=FollowerAxes  RotationSequence=XYX  RotationSequenceAngles=[0 0 0]  RotationSequenceAnglesUnits=deg  RotationMatrix=[1 0 0; 0 1 0; 0 0 1]
  pulley2 : sm_lib/Body Elements/Cylindrical Solid  GraphicAmbientColor=[0.15 0.15 0.15 1.0]  BasedOnType=Mass  CenterOfMass=[0 0 0]  CenterOfMassUnits=m  GraphicDiffuseColor=c.sheave  CylinderLength=P.h  CylinderLengthUnits=mm  CylinderRadius=P.Bd*0.5  CylinderRadiusUnits=mm  Density=0  DensityUnits=kg/m^3  DoExposeReferenceFrame=off  GraphicEmissiveColor=[0.0 0.0 0.0 1.0]  ExportEntireGeometry=off  SerializedFrames=<Frames><Frame><Id>Frame1</Id><Value><Name>F1</Name><Origin><Source>ReferenceFrame</Source><FeatureName></FeatureName></Origin><PrimaryAxis><DefinedDirection>+Z</DefinedDirection><Source>ReferenceFrame</Source><SourceDirection>-Y</SourceDirection><FeatureName></FeatureName></PrimaryAxis><SecondaryAxis><DefinedDirection>+X</DefinedDirection><Source>ReferenceFrame</Source><SourceDirection>+X</SourceDirection><FeatureName></FeatureName></SecondaryAxis></Value></Frame></Frames>  MarkerShape=Frame  MarkerSize=10  GraphicType=FromGeometry  InertiaType=CalculateFromGeometry  Mass=P.Bm/2  MassUnits=kg  MomentsOfInertia=[1 1 1]  MomentsOfInertiaUnits=kg*m^2  GraphicOpacity=1.0  ProductsOfInertia=[0 0 0]  ProductsOfInertiaUnits=kg*m^2  GraphicShininess=10  GraphicSpecularColor=[0.8 0.8 0.8]  GraphicVisPropType=SimpleVisualProperties
  tags : Subsystem  mask{phi0=phi0_shm, s=1}
      mask prompts: phi0 "angle (deg)"; s "direction (1 | -1)"
  F : PMIOPort  Side=Left
  R : PMIOPort  Port=2  Side=Right
  connections:
  R/RConn1 -- tags/LConn1 -- Rigid Transform/RConn1 -- F/RConn1
  pulley2/LConn1 -- Rigid Transform/LConn1

== system DemonstratorSimscape/Transmission System/Roof Pulley Set/Sheave_06/Bending loss ==
  Sin (kN) : Inport
  w (deg/s) : Inport  Port=2
  Add : Sum
  Add1 : Sum  Inputs=+-
  Constant : Constant
  Constant2 : Constant
  Math Function : Math  Operator=pow  SignedPower=on  SaturateOnIntegerOverflow=on
  Product : Product
  Product1 : Product
  Scope : Scope
  dT_Gain : Gain  Gain=-1
  dr for positive omega : Constant
  dr switch : MATLAB Function  TreatAsAtomicUnit=on
  eta_sh : Constant  Value=eta_sh/2
  torque (Nm) : Gain  Gain=r_sheave
  dT (Nm) : Outport  VectorParamsAs1DForOutWhenUnconnected=off
  Sout (kN) : Outport  Port=2  VectorParamsAs1DForOutWhenUnconnected=off
  wires:
  Add/1 -> Math Function/1
  Sin (kN)/1 -> Product1/2, Product/2
  torque (Nm)/1 -> Scope/1, dT_Gain/1
  Math Function/1 -> Add1/1, Product1/1
  Add1/1 -> Product/1
  Product/1 -> torque (Nm)/1
  eta_sh/1 -> Add/2
  Constant/1 -> Add/1
  Constant2/1 -> Add1/2
  Product1/1 -> Sout (kN)/1
  dT_Gain/1 -> dT (Nm)/1
  dr for positive omega/1 -> dr switch/2(dr_wpos)
  dr switch/1(dr) -> Math Function/2
  w (deg/s)/1 -> dr switch/1(w)

== system DemonstratorSimscape/Transmission System/Roof Pulley Set/Sheave_06/PS>Sim1 ==
  b (deg/s^2) : nesl_utility/PS-Simulink Converter  PhysicalDomain=network_engine_domain  SubClassName=ps_output  LeftPortType=input  RightPortType=output  PseudoPeriodic=off  Frequencies=[]  Unit=deg/s^2  AffineConversion=off
  fc (N) : nesl_utility/PS-Simulink Converter  PhysicalDomain=network_engine_domain  SubClassName=ps_output  LeftPortType=input  RightPortType=output  PseudoPeriodic=off  Frequencies=[]  Unit=N  AffineConversion=off
  ft (N) : nesl_utility/PS-Simulink Converter  PhysicalDomain=network_engine_domain  SubClassName=ps_output  LeftPortType=input  RightPortType=output  PseudoPeriodic=off  Frequencies=[]  Unit=N  AffineConversion=off
  q (deg) : nesl_utility/PS-Simulink Converter  PhysicalDomain=network_engine_domain  SubClassName=ps_output  LeftPortType=input  RightPortType=output  PseudoPeriodic=off  Frequencies=[]  Unit=deg  AffineConversion=off
  t (Nm) : nesl_utility/PS-Simulink Converter  PhysicalDomain=network_engine_domain  SubClassName=ps_output  LeftPortType=input  RightPortType=output  PseudoPeriodic=off  Frequencies=[]  Unit=N*m  AffineConversion=off
  tc (Nm) : nesl_utility/PS-Simulink Converter  PhysicalDomain=network_engine_domain  SubClassName=ps_output  LeftPortType=input  RightPortType=output  PseudoPeriodic=off  Frequencies=[]  Unit=N*m  AffineConversion=off
  tt (Nm) : nesl_utility/PS-Simulink Converter  PhysicalDomain=network_engine_domain  SubClassName=ps_output  LeftPortType=input  RightPortType=output  PseudoPeriodic=off  Frequencies=[]  Unit=N*m  AffineConversion=off
  w (deg/s) : nesl_utility/PS-Simulink Converter  PhysicalDomain=network_engine_domain  SubClassName=ps_output  LeftPortType=input  RightPortType=output  PseudoPeriodic=off  Frequencies=[]  Unit=deg/s  AffineConversion=off
  q : PMIOPort  Side=Left
  Conn2 : PMIOPort  Port=2  Side=Left
  Conn3 : PMIOPort  Port=3  Side=Left
  Conn4 : PMIOPort  Port=4  Side=Left
  Conn5 : PMIOPort  Port=5  Side=Left
  Conn6 : PMIOPort  Port=6  Side=Left
  Conn7 : PMIOPort  Port=7  Side=Left
  Conn8 : PMIOPort  Port=8  Side=Left
  Out1 : Outport  VectorParamsAs1DForOutWhenUnconnected=off
  Out2 : Outport  Port=2  VectorParamsAs1DForOutWhenUnconnected=off
  Out3 : Outport  Port=3  VectorParamsAs1DForOutWhenUnconnected=off
  Out4 : Outport  Port=4  VectorParamsAs1DForOutWhenUnconnected=off
  Out5 : Outport  Port=5  VectorParamsAs1DForOutWhenUnconnected=off
  Out6 : Outport  Port=6  VectorParamsAs1DForOutWhenUnconnected=off
  Out7 : Outport  Port=7  VectorParamsAs1DForOutWhenUnconnected=off
  Out8 : Outport  Port=8  VectorParamsAs1DForOutWhenUnconnected=off
  wires:
  q (deg)/1 -> Out1/1
  w (deg/s)/1 -> Out2/1
  b (deg/s^2)/1 -> Out3/1
  t (Nm)/1 -> Out4/1
  fc (N)/1 -> Out5/1
  tc (Nm)/1 -> Out6/1
  ft (N)/1 -> Out7/1
  tt (Nm)/1 -> Out8/1
  connections:
  q/RConn1 -- q (deg)/LConn1
  Conn2/RConn1 -- w (deg/s)/LConn1
  Conn3/RConn1 -- b (deg/s^2)/LConn1
  Conn4/RConn1 -- t (Nm)/LConn1
  fc (N)/LConn1 -- Conn5/RConn1
  Conn6/RConn1 -- tc (Nm)/LConn1
  ft (N)/LConn1 -- Conn7/RConn1
  Conn8/RConn1 -- tt (Nm)/LConn1

== system DemonstratorSimscape/Transmission System/Roof Pulley Set/Sheave_06/Sheave6 ==
  Rigid Transform : sm_lib/Frames and Transforms/Rigid Transform  TranslationMethod=None  TranslationStandardOffset=0  TranslationLengthUnit=m  TranslationStandardAxis=+Z  TranslationCartesianOffset=[0 0 0]  TranslationROffset=0  TranslationROffsetUnits=m  TranslationZOffset=0  TranslationZOffsetUnits=m  TranslationThetaOffset=0  TranslationThetaOffsetUnits=deg  RotationMethod=StandardAxis  RotationAngleUnits=deg  RotationStandardAxis=+X  RotationAngle=90  RotationArbitraryAxis=[0 0 1]  FollAlignAxisA=+X  BaseAlignAxisA=+Y  FollAlignAxisB=+Y  BaseAlignAxisB=+Z  RotationSequenceAxes=FollowerAxes  RotationSequence=XYX  RotationSequenceAngles=[0 0 0]  RotationSequenceAnglesUnits=deg  RotationMatrix=[1 0 0; 0 1 0; 0 0 1]
  pulley2 : sm_lib/Body Elements/Cylindrical Solid  GraphicAmbientColor=[0.15 0.15 0.15 1.0]  BasedOnType=Mass  CenterOfMass=[0 0 0]  CenterOfMassUnits=m  GraphicDiffuseColor=c.sheave  CylinderLength=P.h  CylinderLengthUnits=mm  CylinderRadius=P.d*0.5  CylinderRadiusUnits=mm  Density=0  DensityUnits=kg/m^3  DoExposeReferenceFrame=off  GraphicEmissiveColor=[0.0 0.0 0.0 1.0]  ExportEntireGeometry=off  SerializedFrames=<Frames><Frame><Id>Frame1</Id><Value><Name>F1</Name><Origin><Source>ReferenceFrame</Source><FeatureName></FeatureName></Origin><PrimaryAxis><DefinedDirection>+Z</DefinedDirection><Source>ReferenceFrame</Source><SourceDirection>-Y</SourceDirection><FeatureName></FeatureName></PrimaryAxis><SecondaryAxis><DefinedDirection>+X</DefinedDirection><Source>ReferenceFrame</Source><SourceDirection>+X</SourceDirection><FeatureName></FeatureName></SecondaryAxis></Value></Frame></Frames>  MarkerShape=Frame  MarkerSize=10  GraphicType=FromGeometry  InertiaType=CalculateFromGeometry  Mass=P.m  MassUnits=kg  MomentsOfInertia=[1 1 1]  MomentsOfInertiaUnits=kg*m^2  GraphicOpacity=1.0  ProductsOfInertia=[0 0 0]  ProductsOfInertiaUnits=kg*m^2  GraphicShininess=10  GraphicSpecularColor=[0.8 0.8 0.8]  GraphicVisPropType=SimpleVisualProperties
  tags : Subsystem  mask{phi0=phi0_shm, s=1}
      mask prompts: phi0 "angle (deg)"; s "direction (1 | -1)"
  F : PMIOPort  Side=Left
  R : PMIOPort  Port=2  Side=Right
  connections:
  R/RConn1 -- Rigid Transform/RConn1 -- tags/LConn1 -- F/RConn1
  pulley2/LConn1 -- Rigid Transform/LConn1

== system DemonstratorSimscape/Transmission System/Roof Pulley Set/Sheave_07/Bending loss ==
  Sin (kN) : Inport
  w (deg/s) : Inport  Port=2
  Add : Sum
  Add1 : Sum  Inputs=+-
  Constant : Constant
  Constant2 : Constant
  Math Function : Math  Operator=pow  SignedPower=on  SaturateOnIntegerOverflow=on
  Product : Product
  Product1 : Product
  Scope : Scope
  dT_Gain : Gain  Gain=-1
  dr for positive omega : Constant
  dr switch : MATLAB Function  TreatAsAtomicUnit=on
  eta_sh : Constant  Value=eta_sh/2
  torque (Nm) : Gain  Gain=r_sheave
  dT (Nm) : Outport  VectorParamsAs1DForOutWhenUnconnected=off
  Sout (kN) : Outport  Port=2  VectorParamsAs1DForOutWhenUnconnected=off
  wires:
  Add/1 -> Math Function/1
  Sin (kN)/1 -> Product1/2, Product/2
  torque (Nm)/1 -> Scope/1, dT_Gain/1
  Math Function/1 -> Add1/1, Product1/1
  Add1/1 -> Product/1
  Product/1 -> torque (Nm)/1
  eta_sh/1 -> Add/2
  Constant/1 -> Add/1
  Constant2/1 -> Add1/2
  Product1/1 -> Sout (kN)/1
  dT_Gain/1 -> dT (Nm)/1
  dr for positive omega/1 -> dr switch/2(dr_wpos)
  dr switch/1(dr) -> Math Function/2
  w (deg/s)/1 -> dr switch/1(w)

== system DemonstratorSimscape/Transmission System/Roof Pulley Set/Sheave_07/PS>Sim1 ==
  b (deg/s^2) : nesl_utility/PS-Simulink Converter  PhysicalDomain=network_engine_domain  SubClassName=ps_output  LeftPortType=input  RightPortType=output  PseudoPeriodic=off  Frequencies=[]  Unit=deg/s^2  AffineConversion=off
  fc (N) : nesl_utility/PS-Simulink Converter  PhysicalDomain=network_engine_domain  SubClassName=ps_output  LeftPortType=input  RightPortType=output  PseudoPeriodic=off  Frequencies=[]  Unit=N  AffineConversion=off
  ft (N) : nesl_utility/PS-Simulink Converter  PhysicalDomain=network_engine_domain  SubClassName=ps_output  LeftPortType=input  RightPortType=output  PseudoPeriodic=off  Frequencies=[]  Unit=N  AffineConversion=off
  q (deg) : nesl_utility/PS-Simulink Converter  PhysicalDomain=network_engine_domain  SubClassName=ps_output  LeftPortType=input  RightPortType=output  PseudoPeriodic=off  Frequencies=[]  Unit=deg  AffineConversion=off
  t (Nm) : nesl_utility/PS-Simulink Converter  PhysicalDomain=network_engine_domain  SubClassName=ps_output  LeftPortType=input  RightPortType=output  PseudoPeriodic=off  Frequencies=[]  Unit=N*m  AffineConversion=off
  tc (Nm) : nesl_utility/PS-Simulink Converter  PhysicalDomain=network_engine_domain  SubClassName=ps_output  LeftPortType=input  RightPortType=output  PseudoPeriodic=off  Frequencies=[]  Unit=N*m  AffineConversion=off
  tt (Nm) : nesl_utility/PS-Simulink Converter  PhysicalDomain=network_engine_domain  SubClassName=ps_output  LeftPortType=input  RightPortType=output  PseudoPeriodic=off  Frequencies=[]  Unit=N*m  AffineConversion=off
  w (deg/s) : nesl_utility/PS-Simulink Converter  PhysicalDomain=network_engine_domain  SubClassName=ps_output  LeftPortType=input  RightPortType=output  PseudoPeriodic=off  Frequencies=[]  Unit=deg/s  AffineConversion=off
  q : PMIOPort  Side=Left
  Conn2 : PMIOPort  Port=2  Side=Left
  Conn3 : PMIOPort  Port=3  Side=Left
  Conn4 : PMIOPort  Port=4  Side=Left
  Conn5 : PMIOPort  Port=5  Side=Left
  Conn6 : PMIOPort  Port=6  Side=Left
  Conn7 : PMIOPort  Port=7  Side=Left
  Conn8 : PMIOPort  Port=8  Side=Left
  Out1 : Outport  VectorParamsAs1DForOutWhenUnconnected=off
  Out2 : Outport  Port=2  VectorParamsAs1DForOutWhenUnconnected=off
  Out3 : Outport  Port=3  VectorParamsAs1DForOutWhenUnconnected=off
  Out4 : Outport  Port=4  VectorParamsAs1DForOutWhenUnconnected=off
  Out5 : Outport  Port=5  VectorParamsAs1DForOutWhenUnconnected=off
  Out6 : Outport  Port=6  VectorParamsAs1DForOutWhenUnconnected=off
  Out7 : Outport  Port=7  VectorParamsAs1DForOutWhenUnconnected=off
  Out8 : Outport  Port=8  VectorParamsAs1DForOutWhenUnconnected=off
  wires:
  tt (Nm)/1 -> Out8/1
  ft (N)/1 -> Out7/1
  tc (Nm)/1 -> Out6/1
  fc (N)/1 -> Out5/1
  t (Nm)/1 -> Out4/1
  b (deg/s^2)/1 -> Out3/1
  w (deg/s)/1 -> Out2/1
  q (deg)/1 -> Out1/1
  connections:
  Conn8/RConn1 -- tt (Nm)/LConn1
  ft (N)/LConn1 -- Conn7/RConn1
  Conn6/RConn1 -- tc (Nm)/LConn1
  fc (N)/LConn1 -- Conn5/RConn1
  Conn4/RConn1 -- t (Nm)/LConn1
  Conn3/RConn1 -- b (deg/s^2)/LConn1
  Conn2/RConn1 -- w (deg/s)/LConn1
  q/RConn1 -- q (deg)/LConn1

== system DemonstratorSimscape/Transmission System/Roof Pulley Set/Sheave_07/Sheave7 ==
  Rigid Transform : sm_lib/Frames and Transforms/Rigid Transform  TranslationMethod=None  TranslationStandardOffset=0  TranslationLengthUnit=m  TranslationStandardAxis=+Z  TranslationCartesianOffset=[0 0 0]  TranslationROffset=0  TranslationROffsetUnits=m  TranslationZOffset=0  TranslationZOffsetUnits=m  TranslationThetaOffset=0  TranslationThetaOffsetUnits=deg  RotationMethod=StandardAxis  RotationAngleUnits=deg  RotationStandardAxis=+X  RotationAngle=90  RotationArbitraryAxis=[0 0 1]  FollAlignAxisA=+X  BaseAlignAxisA=+Y  FollAlignAxisB=+Y  BaseAlignAxisB=+Z  RotationSequenceAxes=FollowerAxes  RotationSequence=XYX  RotationSequenceAngles=[0 0 0]  RotationSequenceAnglesUnits=deg  RotationMatrix=[1 0 0; 0 1 0; 0 0 1]
  pulley2 : sm_lib/Body Elements/Cylindrical Solid  GraphicAmbientColor=[0.15 0.15 0.15 1.0]  BasedOnType=Mass  CenterOfMass=[0 0 0]  CenterOfMassUnits=m  GraphicDiffuseColor=c.sheave  CylinderLength=P.h  CylinderLengthUnits=mm  CylinderRadius=P.d*0.5  CylinderRadiusUnits=mm  Density=0  DensityUnits=kg/m^3  DoExposeReferenceFrame=off  GraphicEmissiveColor=[0.0 0.0 0.0 1.0]  ExportEntireGeometry=off  SerializedFrames=<Frames><Frame><Id>Frame1</Id><Value><Name>F1</Name><Origin><Source>ReferenceFrame</Source><FeatureName></FeatureName></Origin><PrimaryAxis><DefinedDirection>+Z</DefinedDirection><Source>ReferenceFrame</Source><SourceDirection>-Y</SourceDirection><FeatureName></FeatureName></PrimaryAxis><SecondaryAxis><DefinedDirection>+X</DefinedDirection><Source>ReferenceFrame</Source><SourceDirection>+X</SourceDirection><FeatureName></FeatureName></SecondaryAxis></Value></Frame></Frames>  MarkerShape=Frame  MarkerSize=10  GraphicType=FromGeometry  InertiaType=CalculateFromGeometry  Mass=P.m  MassUnits=kg  MomentsOfInertia=[1 1 1]  MomentsOfInertiaUnits=kg*m^2  GraphicOpacity=1.0  ProductsOfInertia=[0 0 0]  ProductsOfInertiaUnits=kg*m^2  GraphicShininess=10  GraphicSpecularColor=[0.8 0.8 0.8]  GraphicVisPropType=SimpleVisualProperties
  tags : Subsystem  mask{phi0=phi0_shm, s=1}
      mask prompts: phi0 "angle (deg)"; s "direction (1 | -1)"
  F : PMIOPort  Side=Left
  R : PMIOPort  Port=2  Side=Right
  connections:
  R/RConn1 -- tags/LConn1 -- Rigid Transform/RConn1 -- F/RConn1
  pulley2/LConn1 -- Rigid Transform/LConn1

== system DemonstratorSimscape/Visualization/System Powers/Power and Efficiency/Lumped Efficiency Left ==
  motor speed [rpm] : Inport
  mech power [W] : Inport  Port=2
  Abs1 : Abs
  Constant : Constant  Value=M.eff
  Constant1 : Constant  Value=M.effType
  Constant2 : Constant  Value=M.w
  Constant6 : Constant  Value=VSD.eff
  Divide2 : Product  Inputs=*/
  Divide4 : Product  Inputs=**
  Gain : Gain  Gain=-1
  Gain2 : Gain  Gain=M.eff
  Power : Math  Operator=pow  SaturateOnIntegerOverflow=on
  Product : Product  Inputs=**
  Saturation2 : Saturate  UpperLimit=M.eff  LowerLimit=M.eff*0.5
  Sign : Signum
  Switch : Switch  Criteria=u2 > Threshold  Threshold=0.5
  elec power (W) : Outport  VectorParamsAs1DForOutWhenUnconnected=off
  wires:
  Product/1 -> elec power (W)/1
  motor speed [rpm]/1 -> Gain/1, Abs1/1
  Power/1 -> Product/1
  Divide4/1 -> Power/1
  Abs1/1 -> Gain2/1
  Switch/1 -> Divide4/1
  Constant2/1 -> Divide2/2
  Gain2/1 -> Divide2/1
  Saturation2/1 -> Switch/1
  Constant/1 -> Switch/3
  Constant1/1 -> Switch/2
  Divide2/1 -> Saturation2/1
  Constant6/1 -> Divide4/2
  Gain/1 -> Sign/1
  Sign/1 -> Power/2
  mech power [W]/1 -> Product/2

== system DemonstratorSimscape/Visualization/System Powers/Power and Efficiency/Lumped Efficiency Right ==
  motor speed [rpm] : Inport
  mech power [W] : Inport  Port=2
  Abs1 : Abs
  Constant : Constant  Value=M.eff
  Constant1 : Constant  Value=M.effType
  Constant2 : Constant  Value=M.w
  Constant6 : Constant  Value=VSD.eff
  Divide2 : Product  Inputs=*/
  Divide4 : Product  Inputs=**
  Gain : Gain  Gain=-1
  Gain2 : Gain  Gain=M.eff
  Power : Math  Operator=pow  SaturateOnIntegerOverflow=on
  Product : Product  Inputs=**
  Saturation2 : Saturate  UpperLimit=M.eff  LowerLimit=M.eff*0.5
  Sign : Signum
  Switch : Switch  Criteria=u2 > Threshold  Threshold=0.5
  elec power (W) : Outport  VectorParamsAs1DForOutWhenUnconnected=off
  wires:
  mech power [W]/1 -> Product/2
  Sign/1 -> Power/2
  Gain/1 -> Sign/1
  Constant6/1 -> Divide4/2
  Divide2/1 -> Saturation2/1
  Constant1/1 -> Switch/2
  Constant/1 -> Switch/3
  Saturation2/1 -> Switch/1
  Gain2/1 -> Divide2/1
  Constant2/1 -> Divide2/2
  Switch/1 -> Divide4/1
  Abs1/1 -> Gain2/1
  Divide4/1 -> Power/1
  Power/1 -> Product/1
  motor speed [rpm]/1 -> Abs1/1, Gain/1
  Product/1 -> elec power (W)/1

== system DemonstratorSimscape/EM System/Drives/PLC and Drive Logic Rev3/PLC/1st order LPF1 ==
  Signal : Inport
  Time Constant : Inport  Port=2
  Add1 : Sum
  Add3 : Sum
  Add4 : Sum  Inputs=+-
  Constant1 : Constant  Value=Controller_sampleTime
  Divide : Product  Inputs=*/
  Memory1 : Memory  InitialCondition=Yo  InheritSampleTime=on
  Product1 : Product  RndMeth=Zero
  Signal Out : Outport  VectorParamsAs1DForOutWhenUnconnected=off
  wires:
  Add1/1 -> Divide/2
  Divide/1 -> Product1/1
  Add3/1 -> Memory1/1, Signal Out/1
  Product1/1 -> Add3/2
  Memory1/1 -> Add4/2, Add3/1
  Add4/1 -> Product1/2
  Time Constant/1 -> Add1/2
  Constant1/1 -> Add1/1, Divide/1
  Signal/1 -> Add4/1

== system DemonstratorSimscape/EM System/Drives/PLC and Drive Logic Rev3/PLC/1st order LPF2 ==
  Signal : Inport
  Time Constant : Inport  Port=2
  Add1 : Sum
  Add3 : Sum
  Add4 : Sum  Inputs=+-
  Constant1 : Constant  Value=Controller_sampleTime
  Divide : Product  Inputs=*/
  Memory1 : Memory  InitialCondition=Yo  InheritSampleTime=on
  Product1 : Product  RndMeth=Zero
  Signal Out : Outport  VectorParamsAs1DForOutWhenUnconnected=off
  wires:
  Signal/1 -> Add4/1
  Constant1/1 -> Divide/1, Add1/1
  Time Constant/1 -> Add1/2
  Add4/1 -> Product1/2
  Memory1/1 -> Add3/1, Add4/2
  Product1/1 -> Add3/2
  Add3/1 -> Signal Out/1, Memory1/1
  Divide/1 -> Product1/1
  Add1/1 -> Divide/2
